simulink model "Example_Faulty_DataGen"  (R2022b)
settings: Solver=ode45  StartTime=0.0  StopTime=m_steps  FixedStep=ts  MaxStep=0.1  RelTol=1e-3  EnableMultiTasking=on
values from neighbouring files (symbols this model uses):
  A = 154    [init_model.m]
  a01 = 0.05    [init_model.m]
  a02 = 0.05    [init_model.m]
  attack_time = 70000    [fault_scenario.m]
  az1 = 0.46    [init_model.m]
  az2 = 0.60    (= 0.6)    [init_model.m]
  az3 = 0.45    [init_model.m]
  F_leak1_gain = fault_gain    [fault_scenario.m]    (also in init_model.m = 0)
  F_leak1_time = fault_time    [fault_scenario.m]    (also in init_model.m = 0)
  F_leak2_gain = fault_gain    [fault_scenario.m]    (also in init_model.m = 0)
  F_leak2_time = fault_time    [fault_scenario.m]    (also in init_model.m = 0)
  F_leak3_gain = fault_gain    [fault_scenario.m]    (also in init_model.m = 0)
  F_leak3_time = fault_time    [fault_scenario.m]    (also in init_model.m = 0)
  F_plugg13_gain = fault_gain    [fault_scenario.m]    (also in init_model.m = 0)
  F_plugg13_time = fault_time    [fault_scenario.m]    (also in init_model.m = 0)
  F_plugg20_gain = fault_gain    [fault_scenario.m]    (also in init_model.m = 0)
  F_plugg20_time = fault_time    [fault_scenario.m]    (also in init_model.m = 0)
  F_plugg32_gain = fault_gain    [fault_scenario.m]    (also in init_model.m = 0)
  F_plugg32_time = fault_time    [fault_scenario.m]    (also in init_model.m = 0)
  F_pump1_gain = fault_gain    [fault_scenario.m]    (also in init_model.m = 100)
  F_pump1_time = fault_time    [fault_scenario.m]    (also in init_model.m = 0)
  F_pump2_gain = fault_gain    [fault_scenario.m]    (also in init_model.m = 100)
  F_pump2_time = fault_time    [fault_scenario.m]    (also in init_model.m = 0)
  F_sensor1_offset = fault_gain    [fault_scenario.m]    (also in init_model.m = 0)
  F_sensor1_time = fault_time    [fault_scenario.m]    (also in init_model.m = 0)
  F_sensor2_offset = fault_gain    [fault_scenario.m]    (also in init_model.m = 0)
  F_sensor2_time = fault_time    [fault_scenario.m]    (also in init_model.m = 0)
  F_sensor3_offset = fault_gain    [fault_scenario.m]    (also in init_model.m = 0)
  F_sensor3_time = fault_time    [fault_scenario.m]    (also in init_model.m = 0)
  g = 981    [init_model.m]
  Hmax = 62    [init_model.m]
  l1 = a01    (= 0.05)    [init_model.m]
  l2 = a02    (= 0.05)    [init_model.m]
  m_ramp1 = 3e-4    (= 0.0003)    [fault_scenario.m]
  m_ramp2 = 0    [fault_scenario.m]
  m_satu = 1    [fault_scenario.m]
  m_satu1 = 460    [fault_scenario.m]
  m_satu2 = 160    [fault_scenario.m]
  m_satu3 = 320    [fault_scenario.m]
  m_ts = 2    [init_model.m]
  m_var1 = 0.2027    [init_model.m]
  m_var2 = 0.4394    [init_model.m]
  m_var3 = 0.0051    [init_model.m]
  p = s    [Att.m]    (also in init_model.m = 0)
  Q1max = 100    [init_model.m]
  Q2max = 100    [init_model.m]
  Sl = 0.5    [init_model.m]
  Sn = 0.5    [init_model.m]
  T_attack = 1000/(2*pi)    (= 159.154943092)    [fault_scenario.m]
  v = k    (= 0.0125)    [init_model.m]
libraries: simulink x5
settings Model: Creator=luo  LastModifiedBy=DaiQi Yang
settings SolverCC: AlgebraicLoopSolver=TrustRegion
settings DataIOCC: LimitDataPoints=on  SaveFormat=Array  SignalLoggingSaveFormat=ModelDataLogs  ReturnWorkspaceOutputs=off
settings OptimizationCC: ReuseModelBlockBuffer=on  ExpressionDepthLimit=2147483647  LifeSpan=inf
settings DebuggingCC: UnderspecifiedInitializationDetection=Classic  MergeDetectMultiDrivingBlocksExec=none  SolverPrmCheckMsg=warning  FcnCallInpInsideContextMsg=warning  UnconnectedInputMsg=warning  UnconnectedOutputMsg=warning  UnconnectedLineMsg=warning  StateNameClashWarn=warning  SFUnexpectedBacktrackingDiag=warning  SFNoUnconditionalDefaultTransitionDiag=warning  SFExecutionAtInitializationDiag=none  ArithmeticOperatorsInVariantConditions=warning
settings HardwareCC: ProdBitPerPointer=32  ProdBitPerSizeT=32  ProdBitPerPtrDiffT=32  ProdLargestAtomicFloat=None  ProdIntDivRoundTo=Undefined  ProdEndianess=Unspecified  ProdWordSize=32  ProdHWDeviceType=32-bit Generic
settings ModelReferenceCC: EnableRefExpFcnMdlSchedulingChecks=on  PropagateSignalLabelsOutOfModel=off
settings SFSimCC: SimUseLocalCustomCode=off  CustomCodeUndefinedFunction=UseInterfaceOnly
settings RTWCC: RTWUseLocalCustomCode=off
settings CodeAppCC: StateflowObjectComments=on
settings GRTTargetCC: TargetLangStandard=C89/C90 (ANSI)  CombineOutputUpdateFcns=off  GRTInterface=on
settings ConfigComp: CovMetricSettings=dw  CovSaveCumulativeToWorkspaceVar=on  CovSaveSingleToWorkspaceVar=on  CovExternalEMLEnable=off

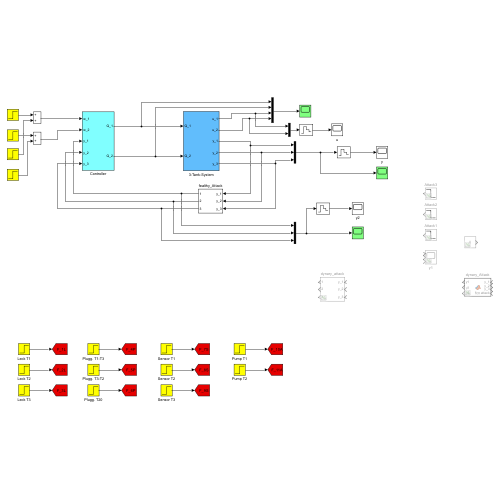
[thumbnail: Simulink's stored preview of the top-level diagram]
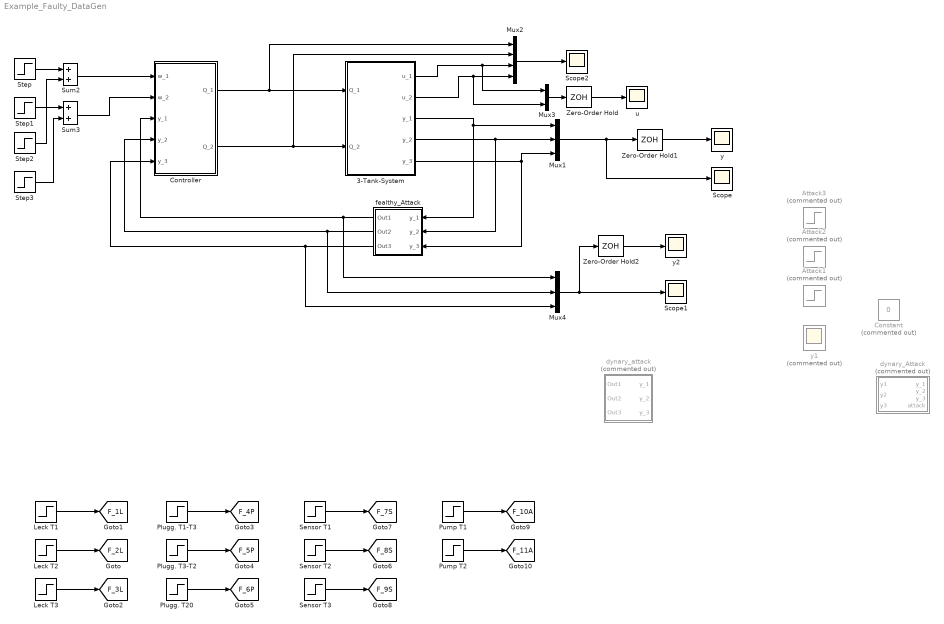
== system Example_Faulty_DataGen ==
  3-Tank-System : Subsystem
  Attack1 : Step  Commented=on  Time=attack_time  After=-0.352325574028282  SampleTime=0
  Attack2 : Step  Commented=on  Time=attack_time  After=-0.352325574028282  SampleTime=0
  Attack3 : Step  Commented=on  Time=attack_time  After=-0.352325574028282  SampleTime=0
  Constant : Constant  Commented=on  Value=0
  Controller : Subsystem
  Leck T1 : Step  Time=F_leak1_time  After=F_leak1_gain  SampleTime=0
  Leck T2 : Step  Time=F_leak2_time  After=F_leak2_gain  SampleTime=0
  Leck T3 : Step  Time=F_leak3_time  After=F_leak3_gain  SampleTime=0
  Mux1 : Mux  Inputs=3
  Mux2 : Mux
  Mux3 : Mux  Inputs=2
  Mux4 : Mux  Inputs=3
  Plugg. T1-T3 : Step  Time=F_plugg13_time  After=F_plugg13_gain  SampleTime=0
  Plugg. T20 : Step  Time=F_plugg20_time  After=F_plugg20_gain  SampleTime=0
  Plugg. T3-T2 : Step  Time=F_plugg32_time  After=F_plugg32_gain  SampleTime=0
  Pump T1 : Step  Time=F_pump1_time  Before=100  After=F_pump1_gain  SampleTime=0
  Pump T2 : Step  Time=F_pump2_time  Before=100  After=F_pump2_gain  SampleTime=0
  Scope : Scope
  Scope1 : Scope
  Scope2 : Scope
  Sensor T1 : Step  Time=500  Before=100  After=100  SampleTime=0
  Sensor T2 : Step  Time=500  Before=100  After=100  SampleTime=0
  Sensor T3 : Step  Time=500  Before=100  After=100  SampleTime=0
  Step : Step  Time=0  After=45  SampleTime=0
  Step1 : Step  Time=0  After=15  SampleTime=0
  Step2 : Step  Time=500  After=0  SampleTime=0
  Step3 : Step  Time=800  After=0  SampleTime=0
  Sum2 : Sum  SaturateOnIntegerOverflow=on
  Sum3 : Sum  SaturateOnIntegerOverflow=on
  Zero-Order Hold : ZeroOrderHold  SampleTime=m_ts
  Zero-Order Hold1 : ZeroOrderHold  SampleTime=m_ts
  Zero-Order Hold2 : ZeroOrderHold  SampleTime=m_ts
  dynary_Attack : MATLAB Function  Commented=on  TreatAsAtomicUnit=on
  dynary_attack : Subsystem  Commented=on
  fealthy_Attack : Subsystem
  u : Scope
  y : Scope
  y1 : Scope  Commented=on  NumInputPorts=3
  y2 : Scope
  tag scope: F_10A=global, F_11A=global, F_1L=global, F_2L=global, F_3L=global, F_4P=global, F_5P=global, F_6P=global, F_7S=global, F_8S=global, F_9S=global
  wires:
  Step/1 -> Sum2/1
  Step1/1 -> Sum3/1
  Step2/1 -> Sum2/2
  Step3/1 -> Sum3/2
  Mux1/1 -> Scope/1, Zero-Order Hold1/1
  Leck T2/1 -> [F_2L]
  Sum2/1 -> Controller/1(w_1)
  Leck T1/1 -> [F_1L]
  Leck T3/1 -> [F_3L]
  Plugg. T1-T3/1 -> [F_4P]
  Plugg. T3-T2/1 -> [F_5P]
  Plugg. T20/1 -> [F_6P]
  Sensor T2/1 -> [F_8S]
  Sensor T1/1 -> [F_7S]
  Sensor T3/1 -> [F_9S]
  Pump T1/1 -> [F_10A]
  Pump T2/1 -> [F_11A]
  Mux2/1 -> Scope2/1
  3-Tank-System/1(u_1) -> Mux3/1, Mux2/3
  3-Tank-System/2(u_2) -> Mux3/2, Mux2/4
  Controller/1(Q_1) -> 3-Tank-System/1(Q_1), Mux2/1
  Controller/2(Q_2) -> 3-Tank-System/2(Q_2), Mux2/2
  Sum3/1 -> Controller/2(w_2)
  Zero-Order Hold/1 -> u/1
  Zero-Order Hold1/1 -> y/1
  Mux3/1 -> Zero-Order Hold/1
  3-Tank-System/3(y_1) -> fealthy_Attack/1(y_1), Mux1/1
  3-Tank-System/4(y_2) -> fealthy_Attack/2(y_2), Mux1/2
  3-Tank-System/5(y_3) -> fealthy_Attack/3(y_3), Mux1/3
  fealthy_Attack/1(Out1) -> Mux4/1, Controller/3(y_1)
  fealthy_Attack/2(Out2) -> Mux4/2, Controller/4(y_2)
  fealthy_Attack/3(Out3) -> Mux4/3, Controller/5(y_3)
  Mux4/1 -> Scope1/1, Zero-Order Hold2/1
  Zero-Order Hold2/1 -> y2/1

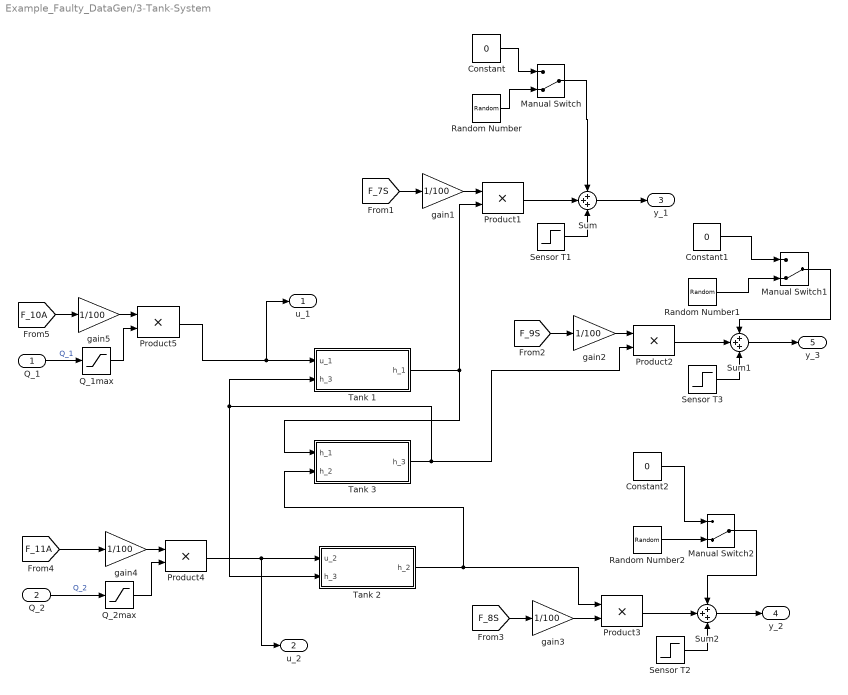
== system Example_Faulty_DataGen/3-Tank-System ==
  Q_1 : Inport
  Q_2 : Inport  Port=2
  Constant : Constant  Value=0
  Constant1 : Constant  Value=0
  Constant2 : Constant  Value=0
  Manual Switch : ManualSwitch  CurrentSetting=0
  Manual Switch1 : ManualSwitch  CurrentSetting=0
  Manual Switch2 : ManualSwitch  CurrentSetting=0
  Product{1..5} (5 alike) : Product  SaturateOnIntegerOverflow=on  OutDataTypeStr=Inherit: Same as first input
  Q_1max : Saturate  UpperLimit=Q1max  LowerLimit=0
  Q_2max : Saturate  UpperLimit=Q2max  LowerLimit=0
  Random Number : RandomNumber  Variance=m_var1  Seed=floor(1000*rand(1))  SampleTime=0
  Random Number1 : RandomNumber  Variance=m_var3  Seed=floor(1000*rand(1))  SampleTime=0
  Random Number2 : RandomNumber  Variance=m_var2  Seed=floor(1000*rand(1))  SampleTime=0
  Sensor T1 : Step  Time=F_sensor1_time  After=F_sensor1_offset  SampleTime=0
  Sensor T2 : Step  Time=F_sensor2_time  After=F_sensor2_offset  SampleTime=0
  Sensor T3 : Step  Time=F_sensor3_time  After=F_sensor3_offset  SampleTime=0
  Sum : Sum  Inputs=+++
  Sum1 : Sum  Inputs=+++
  Sum2 : Sum  Inputs=+++
  Tank 1 : Subsystem
  Tank 2 : Subsystem
  Tank 3 : Subsystem
  gain{1..5} (5 alike) : Gain  Gain=1/100  SaturateOnIntegerOverflow=on  OutDataTypeStr=Inherit: Same as input  ParamDataTypeStr=Inherit: Same as input
  u_1 : Outport  VectorParamsAs1DForOutWhenUnconnected=off
  u_2 : Outport  Port=2  VectorParamsAs1DForOutWhenUnconnected=off
  y_1 : Outport  Port=3  VectorParamsAs1DForOutWhenUnconnected=off
  y_2 : Outport  Port=4  VectorParamsAs1DForOutWhenUnconnected=off
  y_3 : Outport  Port=5  VectorParamsAs1DForOutWhenUnconnected=off
  wires:
  Tank 1/1(h_1) -> Tank 3/1(h_1), Product1/2
  Tank 3/1(h_3) -> Tank 1/2(h_3), Tank 2/2(h_3), Product2/2
  Tank 2/1(h_2) -> Tank 3/2(h_2), Product3/1
  [F_8S] -> gain3/1
  gain3/1 -> Product3/2
  gain1/1 -> Product1/1
  [F_7S] -> gain1/1
  gain2/1 -> Product2/1
  [F_9S] -> gain2/1
  gain4/1 -> Product4/1
  [F_11A] -> gain4/1
  Q_2/1 -> Q_2max/1  "Q_2"
  Product4/1 -> Tank 2/1(u_2), u_2/1
  gain5/1 -> Product5/1
  [F_10A] -> gain5/1
  Q_1/1 -> Q_1max/1  "Q_1"
  Product5/1 -> Tank 1/1(u_1), u_1/1
  Q_1max/1 -> Product5/2
  Q_2max/1 -> Product4/2
  Product1/1 -> Sum/2
  Sum/1 -> y_1/1
  Product2/1 -> Sum1/2
  Sum1/1 -> y_3/1
  Product3/1 -> Sum2/2
  Sum2/1 -> y_2/1
  Sensor T1/1 -> Sum/3
  Sensor T2/1 -> Sum2/3
  Sensor T3/1 -> Sum1/3
  Constant/1 -> Manual Switch/1
  Random Number/1 -> Manual Switch/2
  Manual Switch/1 -> Sum/1
  Random Number2/1 -> Manual Switch2/2
  Manual Switch2/1 -> Sum2/1
  Random Number1/1 -> Manual Switch1/2
  Manual Switch1/1 -> Sum1/1
  Constant1/1 -> Manual Switch1/1
  Constant2/1 -> Manual Switch2/1

== system Example_Faulty_DataGen/Controller ==
  w_1 : Inport
  w_2 : Inport  Port=2
  y_1 : Inport  Port=3
  y_2 : Inport  Port=4
  y_3 : Inport  Port=5
  Matrix F : Subsystem
  Matrix G : Subsystem
  PI controller 1 : Subsystem
  PI controller 2 : Subsystem
  Sum : Sum  Inputs=|+-
  Sum1 : Sum  Inputs=|+-
  Sum4 : Sum  SaturateOnIntegerOverflow=on
  Sum5 : Sum  SaturateOnIntegerOverflow=on
  Q_1 : Outport  VectorParamsAs1DForOutWhenUnconnected=off
  Q_2 : Outport  Port=2  VectorParamsAs1DForOutWhenUnconnected=off
  wires:
  Sum/1 -> PI controller 1/1(In1)
  Sum1/1 -> PI controller 2/1(In1)
  Matrix F/1(F_2) -> Sum4/2
  Matrix F/2(F_1) -> Sum5/2
  Matrix G/1(G_1) -> Sum5/1
  Matrix G/2(G_2) -> Sum4/1
  PI controller 1/1(Out1) -> Matrix G/1(w_1)
  PI controller 2/1(Out1) -> Matrix G/2(w_2)
  y_3/1 -> Matrix F/3(y_3)
  w_1/1 -> Sum/1
  Sum5/1 -> Q_1/1
  w_2/1 -> Sum1/1
  Sum4/1 -> Q_2/1
  y_2/1 -> Sum1/2, Matrix F/2(y_2)
  y_1/1 -> Matrix F/1(y_1), Sum/2

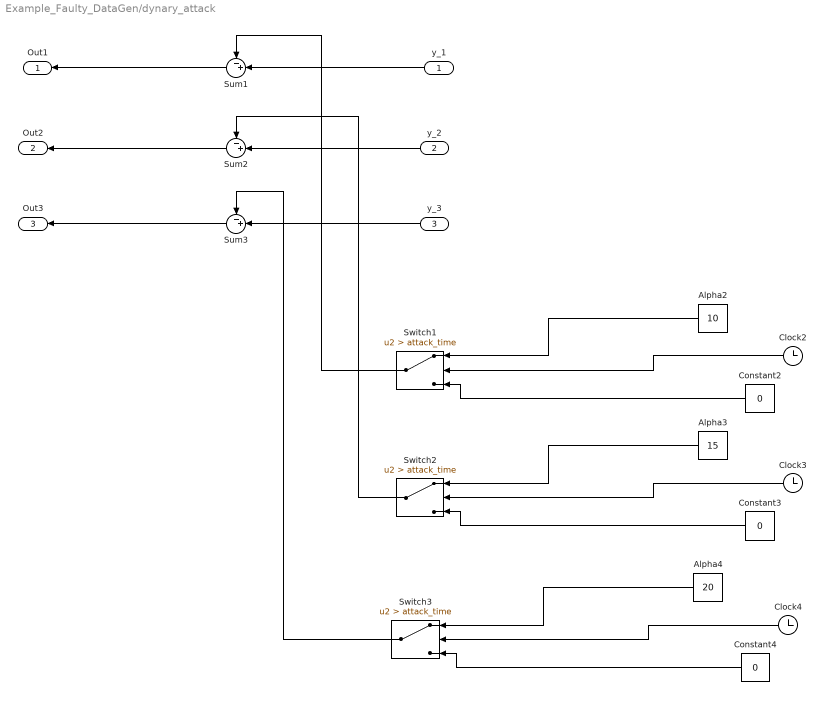
== system Example_Faulty_DataGen/dynary_attack ==
  y_1 : Inport
  y_2 : Inport  Port=2
  y_3 : Inport  Port=3
  Alpha2 : Constant  Value=10
  Alpha3 : Constant  Value=15
  Alpha4 : Constant  Value=20
  Clock2 : Clock
  Clock3 : Clock
  Clock4 : Clock
  Constant2 : Constant  Value=0
  Constant3 : Constant  Value=0
  Constant4 : Constant  Value=0
  Sum1 : Sum  Inputs=-+|
  Sum2 : Sum  Inputs=-+|
  Sum3 : Sum  Inputs=-+|
  Switch1 : Switch  Criteria=u2 > Threshold  Threshold=attack_time  SaturateOnIntegerOverflow=off  InputSameDT=off
  Switch2 : Switch  Criteria=u2 > Threshold  Threshold=attack_time  SaturateOnIntegerOverflow=off  InputSameDT=off
  Switch3 : Switch  Criteria=u2 > Threshold  Threshold=attack_time  SaturateOnIntegerOverflow=off  InputSameDT=off
  Out1 : Outport
  Out2 : Outport  Port=2
  Out3 : Outport  Port=3
  wires:
  Sum1/1 -> Out1/1
  y_1/1 -> Sum1/2
  Clock2/1 -> Switch1/2
  Constant2/1 -> Switch1/3
  Alpha2/1 -> Switch1/1
  Alpha3/1 -> Switch2/1
  Clock3/1 -> Switch2/2
  Constant3/1 -> Switch2/3
  Alpha4/1 -> Switch3/1
  Switch3/1 -> Sum3/1
  Clock4/1 -> Switch3/2
  Constant4/1 -> Switch3/3
  Sum2/1 -> Out2/1
  y_2/1 -> Sum2/2
  Sum3/1 -> Out3/1
  y_3/1 -> Sum3/2
  Switch1/1 -> Sum1/1
  Switch2/1 -> Sum2/1

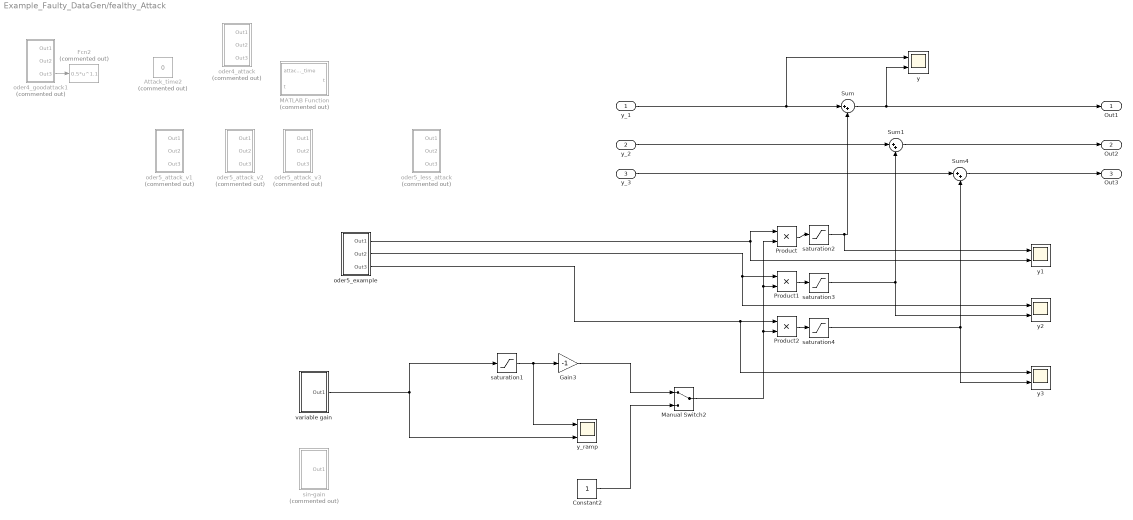
== system Example_Faulty_DataGen/fealthy_Attack ==
  y_1 : Inport
  y_2 : Inport  Port=2
  y_3 : Inport  Port=3
  Attack_time2 : Constant  Commented=on  Value=0
  Constant2 : Constant
  Fcn2 : Fcn  Commented=on  Expr=0.5*u^1.1
  Gain3 : Gain  Gain=-1
  MATLAB Function : MATLAB Function  Commented=on  TreatAsAtomicUnit=on
  Manual Switch2 : ManualSwitch
  Product : Product
  Product1 : Product
  Product2 : Product
  Sum : Sum  Inputs=|++
  Sum1 : Sum  Inputs=|++
  Sum4 : Sum  Inputs=|++
  oder4_attack : Subsystem  Commented=on
  oder4_goodattack1 : Subsystem  Commented=on
  oder5_attack_v1 : Subsystem  Commented=on
  oder5_attack_v2 : Subsystem  Commented=on
  oder5_attack_v3 : Subsystem  Commented=on
  oder5_example : Subsystem
  oder5_less_attack : Subsystem  Commented=on
  saturation1 : Saturate  UpperLimit=m_satu  LowerLimit=-m_satu
  saturation2 : Saturate  UpperLimit=m_satu1  LowerLimit=-m_satu1
  saturation3 : Saturate  UpperLimit=m_satu2  LowerLimit=-m_satu2
  saturation4 : Saturate  UpperLimit=m_satu3  LowerLimit=-m_satu3
  sin-gain : Subsystem  Commented=on
  variable gain : Subsystem
  y{,1..3} (4 alike) : Scope  NumInputPorts=2
  y_ramp : Scope  NumInputPorts=2
  Out1 : Outport
  Out2 : Outport  Port=2
  Out3 : Outport  Port=3
  wires:
  Sum/1 -> y/2, Out1/1
  y_1/1 -> y/1, Sum/1
  Sum4/1 -> Out3/1
  Sum1/1 -> Out2/1
  y_3/1 -> Sum4/1
  y_2/1 -> Sum1/1
  Product/1 -> saturation2/1
  saturation1/1 -> y_ramp/1, Gain3/1
  Constant2/1 -> Manual Switch2/2
  Manual Switch2/1 -> Product2/2, Product1/2, Product/2
  Gain3/1 -> Manual Switch2/1
  saturation2/1 -> y1/1, Sum/2
  Product1/1 -> saturation3/1
  saturation3/1 -> y2/2, Sum1/2
  Product2/1 -> saturation4/1
  saturation4/1 -> Sum4/2, y3/2
  oder5_example/1(Out1) -> y1/2, Product/1
  oder5_example/2(Out2) -> y2/1, Product1/1
  oder5_example/3(Out3) -> y3/1, Product2/1
  variable gain/1(Out1) -> saturation1/1, y_ramp/2
  oder4_goodattack1/3(Out3) -> Fcn2/1

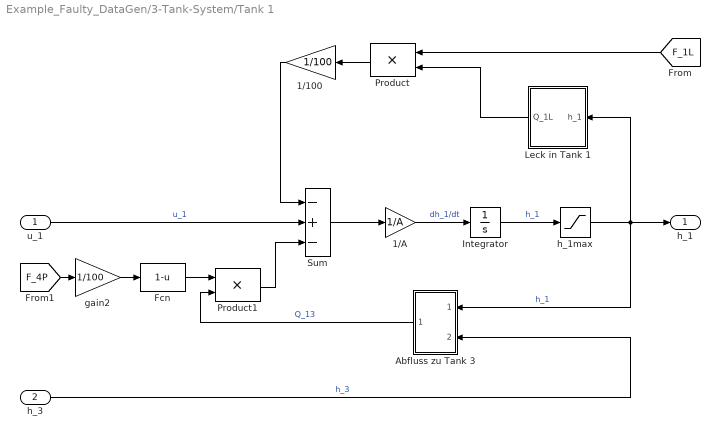
== system Example_Faulty_DataGen/3-Tank-System/Tank 1 ==
  u_1 : Inport
  h_3 : Inport  Port=2
  1/100 : Gain  Gain=1/100  SaturateOnIntegerOverflow=on  OutDataTypeStr=Inherit: Same as input  ParamDataTypeStr=Inherit: Same as input
  1/A : Gain  Gain=1/A  SaturateOnIntegerOverflow=on  OutDataTypeStr=Inherit: Same as input  ParamDataTypeStr=Inherit: Same as input
  Abfluss zu Tank 3 : Subsystem
  Fcn : Fcn  Expr=1-u
  Integrator : Integrator  InitialCondition=0.3
  Leck in Tank 1 : Subsystem
  Product : Product  SaturateOnIntegerOverflow=on  OutDataTypeStr=Inherit: Same as first input
  Product1 : Product  SaturateOnIntegerOverflow=on  OutDataTypeStr=Inherit: Same as first input
  Sum : Sum  Inputs=-+-  SaturateOnIntegerOverflow=on
  gain2 : Gain  Gain=1/100  SaturateOnIntegerOverflow=on  OutDataTypeStr=Inherit: Same as input  ParamDataTypeStr=Inherit: Same as input
  h_1max : Saturate  UpperLimit=Hmax  LowerLimit=0
  h_1 : Outport  VectorParamsAs1DForOutWhenUnconnected=off
  wires:
  1/A/1 -> Integrator/1  "dh_1/dt"
  h_1max/1 -> Abfluss zu Tank 3/1(h_1), Leck in Tank 1/1(h_1), h_1/1  "h_1"
  Integrator/1 -> h_1max/1  "h_1"
  Sum/1 -> 1/A/1
  h_3/1 -> Abfluss zu Tank 3/2(h_3)  "h_3"
  Product/1 -> 1/100/1
  [F_1L] -> Product/1
  Product1/1 -> Sum/3
  Abfluss zu Tank 3/1(Q_13) -> Product1/2  "Q_13"
  1/100/1 -> Sum/1
  Leck in Tank 1/1(Q_1L) -> Product/2
  gain2/1 -> Fcn/1
  [F_4P] -> gain2/1
  Fcn/1 -> Product1/1
  u_1/1 -> Sum/2  "u_1"

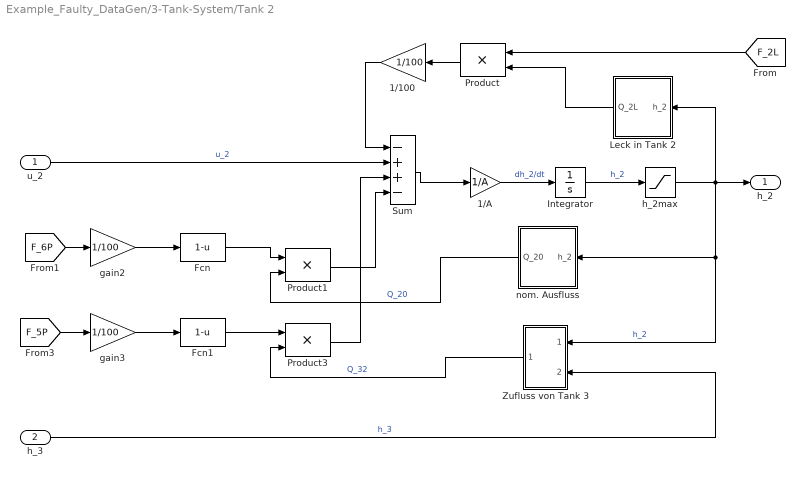
== system Example_Faulty_DataGen/3-Tank-System/Tank 2 ==
  u_2 : Inport
  h_3 : Inport  Port=2
  1/100 : Gain  Gain=1/100  SaturateOnIntegerOverflow=on  OutDataTypeStr=Inherit: Same as input  ParamDataTypeStr=Inherit: Same as input
  1/A : Gain  Gain=1/A  SaturateOnIntegerOverflow=on  OutDataTypeStr=Inherit: Same as input  ParamDataTypeStr=Inherit: Same as input
  Fcn : Fcn  Expr=1-u
  Fcn1 : Fcn  Expr=1-u
  Integrator : Integrator  InitialCondition=0.2
  Leck in Tank 2 : Subsystem
  Product : Product  SaturateOnIntegerOverflow=on  OutDataTypeStr=Inherit: Same as first input
  Product1 : Product  SaturateOnIntegerOverflow=on  OutDataTypeStr=Inherit: Same as first input
  Product3 : Product  SaturateOnIntegerOverflow=on  OutDataTypeStr=Inherit: Same as first input
  Sum : Sum  Inputs=-++-  SaturateOnIntegerOverflow=on
  Zufluss von Tank 3 : Subsystem
  gain2 : Gain  Gain=1/100  SaturateOnIntegerOverflow=on  OutDataTypeStr=Inherit: Same as input  ParamDataTypeStr=Inherit: Same as input
  gain3 : Gain  Gain=1/100  SaturateOnIntegerOverflow=on  OutDataTypeStr=Inherit: Same as input  ParamDataTypeStr=Inherit: Same as input
  h_2max : Saturate  UpperLimit=Hmax  LowerLimit=0
  nom. Ausfluss : Subsystem
  h_2 : Outport  VectorParamsAs1DForOutWhenUnconnected=off
  wires:
  1/A/1 -> Integrator/1  "dh_2/dt"
  h_2max/1 -> nom. Ausfluss/1(h_2), Zufluss von Tank 3/1(h_1), Leck in Tank 2/1(h_2), h_2/1  "h_2"
  Integrator/1 -> h_2max/1  "h_2"
  Sum/1 -> 1/A/1
  h_3/1 -> Zufluss von Tank 3/2(h_3)  "h_3"
  Product/1 -> 1/100/1
  [F_2L] -> Product/1
  1/100/1 -> Sum/1
  Leck in Tank 2/1(Q_2L) -> Product/2
  gain2/1 -> Fcn/1
  [F_6P] -> gain2/1
  gain3/1 -> Fcn1/1
  [F_5P] -> gain3/1
  nom. Ausfluss/1(Q_20) -> Product1/2  "Q_20"
  Product1/1 -> Sum/4
  Zufluss von Tank 3/1(Q_32) -> Product3/2  "Q_32"
  Product3/1 -> Sum/3
  Fcn/1 -> Product1/1
  Fcn1/1 -> Product3/1
  u_2/1 -> Sum/2  "u_2"

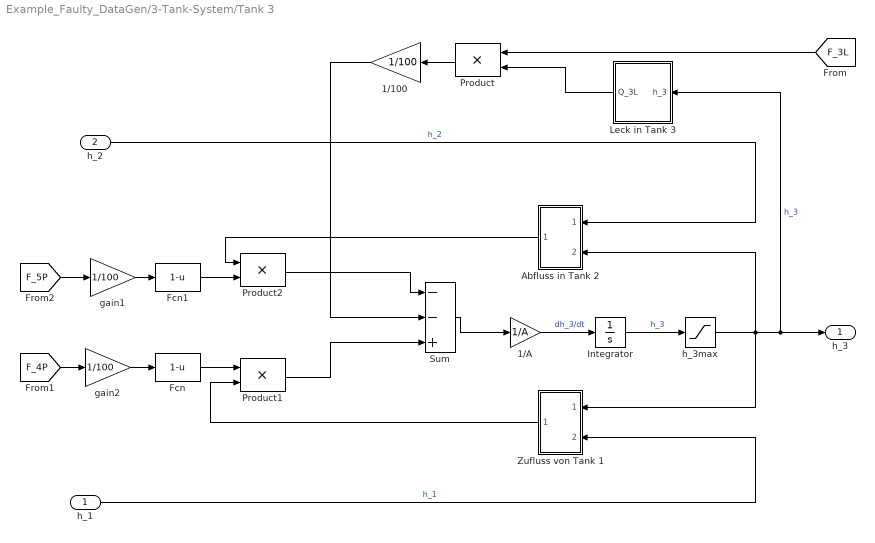
== system Example_Faulty_DataGen/3-Tank-System/Tank 3 ==
  h_1 : Inport
  h_2 : Inport  Port=2
  1/100 : Gain  Gain=1/100  SaturateOnIntegerOverflow=on  OutDataTypeStr=Inherit: Same as input  ParamDataTypeStr=Inherit: Same as input
  1/A : Gain  Gain=1/A  SaturateOnIntegerOverflow=on  OutDataTypeStr=Inherit: Same as input  ParamDataTypeStr=Inherit: Same as input
  Abfluss in Tank 2 : Subsystem
  Fcn : Fcn  Expr=1-u
  Fcn1 : Fcn  Expr=1-u
  Integrator : Integrator  InitialCondition=0.25
  Leck in Tank 3 : Subsystem
  Product : Product  SaturateOnIntegerOverflow=on  OutDataTypeStr=Inherit: Same as first input
  Product1 : Product  SaturateOnIntegerOverflow=on  OutDataTypeStr=Inherit: Same as first input
  Product2 : Product  SaturateOnIntegerOverflow=on  OutDataTypeStr=Inherit: Same as first input
  Sum : Sum  Inputs=--+  SaturateOnIntegerOverflow=on
  Zufluss von Tank 1 : Subsystem
  gain1 : Gain  Gain=1/100  SaturateOnIntegerOverflow=on  OutDataTypeStr=Inherit: Same as input  ParamDataTypeStr=Inherit: Same as input
  gain2 : Gain  Gain=1/100  SaturateOnIntegerOverflow=on  OutDataTypeStr=Inherit: Same as input  ParamDataTypeStr=Inherit: Same as input
  h_3max : Saturate  UpperLimit=Hmax  LowerLimit=0
  h_3 : Outport  VectorParamsAs1DForOutWhenUnconnected=off
  wires:
  1/A/1 -> Integrator/1  "dh_3/dt"
  h_3max/1 -> Abfluss in Tank 2/2(h_3), Zufluss von Tank 1/1(h_3), h_3/1, Leck in Tank 3/1(h_3)  "h_3"
  Integrator/1 -> h_3max/1  "h_3"
  Sum/1 -> 1/A/1
  h_1/1 -> Zufluss von Tank 1/2(h_1)  "h_1"
  h_2/1 -> Abfluss in Tank 2/1(h_2)  "h_2"
  Product/1 -> 1/100/1
  [F_3L] -> Product/1
  gain2/1 -> Fcn/1
  [F_4P] -> gain2/1
  [F_5P] -> gain1/1
  1/100/1 -> Sum/2
  Leck in Tank 3/1(Q_3L) -> Product/2
  Abfluss in Tank 2/1(Q_32) -> Product2/1
  gain1/1 -> Fcn1/1
  Product2/1 -> Sum/1
  Zufluss von Tank 1/1(Q_13) -> Product1/2
  Product1/1 -> Sum/3
  Fcn/1 -> Product1/1
  Fcn1/1 -> Product2/2

== system Example_Faulty_DataGen/Controller/Matrix F ==
  y_1 : Inport
  y_2 : Inport  Port=2
  y_3 : Inport  Port=3
  Abfluss in Tank 2 : Subsystem
  Abfluss zu Tank 3 : Subsystem
  Gain : Gain  Gain=A*a01  SaturateOnIntegerOverflow=on  OutDataTypeStr=Inherit: Same as input  ParamDataTypeStr=Inherit: Same as input
  Gain2 : Gain  Gain=A*a02  SaturateOnIntegerOverflow=on  OutDataTypeStr=Inherit: Same as input  ParamDataTypeStr=Inherit: Same as input
  Sum : Sum  Inputs=-+-  SaturateOnIntegerOverflow=on
  Sum1 : Sum  Inputs=-+  SaturateOnIntegerOverflow=on
  nom. Ausfluss : Subsystem
  F_2 : Outport  VectorParamsAs1DForOutWhenUnconnected=off
  F_1 : Outport  Port=2  VectorParamsAs1DForOutWhenUnconnected=off
  wires:
  y_1/1 -> Abfluss zu Tank 3/1(h_1), Gain/1
  y_3/1 -> Abfluss in Tank 2/1(h_3), Abfluss zu Tank 3/2(h_3)
  y_2/1 -> nom. Ausfluss/1(h_2), Abfluss in Tank 2/2(h_2), Gain2/1
  Sum1/1 -> F_1/1
  Gain/1 -> Sum1/1
  Abfluss zu Tank 3/1(Q_13) -> Sum1/2
  Abfluss in Tank 2/1(Q_32) -> Sum/1
  nom. Ausfluss/1(Q_20) -> Sum/2
  Gain2/1 -> Sum/3
  Sum/1 -> F_2/1

== system Example_Faulty_DataGen/Controller/Matrix G ==
  w_1 : Inport
  w_2 : Inport  Port=2
  Gain 1 : Gain  Gain=A*l1
  Gain 2 : Gain  Gain=A*l2
  G_1 : Outport  VectorParamsAs1DForOutWhenUnconnected=off
  G_2 : Outport  Port=2  VectorParamsAs1DForOutWhenUnconnected=off
  wires:
  w_1/1 -> Gain 1/1
  Gain 1/1 -> G_1/1
  w_2/1 -> Gain 2/1
  Gain 2/1 -> G_2/1

== system Example_Faulty_DataGen/Controller/PI controller 1 ==
  In1 : Inport
  Int1 : Integrator  InitialCondition=0.4
  P1 : Gain  Gain=p
  Sum : Sum  Inputs=|++
  v=k : Gain  Gain=v
  Out1 : Outport  VectorParamsAs1DForOutWhenUnconnected=off
  wires:
  In1/1 -> v=k/1
  P1/1 -> Sum/2
  Int1/1 -> Sum/1
  Sum/1 -> Out1/1
  v=k/1 -> P1/1, Int1/1

== system Example_Faulty_DataGen/Controller/PI controller 2 ==
  In1 : Inport
  Int1 : Integrator  InitialCondition=0.2
  P1 : Gain  Gain=p
  Sum : Sum  Inputs=|++
  v=k : Gain  Gain=v
  Out1 : Outport  VectorParamsAs1DForOutWhenUnconnected=off
  wires:
  In1/1 -> v=k/1
  P1/1 -> Sum/2
  Int1/1 -> Sum/1
  Sum/1 -> Out1/1
  v=k/1 -> P1/1, Int1/1

== system Example_Faulty_DataGen/fealthy_Attack/oder4_attack ==
  Attack1 : Polyval  Coefs=|
      | [0.0147
      | -0.3439
      | 2.7873
      | -9.1137
      | 6.0715]
  Attack2 : Polyval  Coefs=|
      | [0.0187
      | -0.4361
      | 3.5079
      | -11.3885
      | 11.0519]
  Attack3 : Polyval  Coefs=|
      | [-0.0713
      | 1.6694
      | -13.5181
      | 44.1571
      | -50.2598]
  Attack_time : Constant  Value=attack_time
  Clock1 : Clock
  Clock2 : Clock
  Constant1 : Constant  Value=0
  Fcn3 : Fcn  Expr=rem(u,8)+2
  Sum2 : Sum  Inputs=-+|
  Switch : Switch  Criteria=u2 > Threshold  Threshold=attack_time  SaturateOnIntegerOverflow=off  InputSameDT=off
  Out1 : Outport
  Out2 : Outport  Port=2
  Out3 : Outport  Port=3
  wires:
  Fcn3/1 -> Attack3/1, Attack2/1, Attack1/1
  Constant1/1 -> Switch/3
  Clock1/1 -> Switch/2
  Clock2/1 -> Sum2/2
  Attack_time/1 -> Sum2/1
  Sum2/1 -> Switch/1
  Attack3/1 -> Out3/1
  Attack1/1 -> Out1/1
  Attack2/1 -> Out2/1
  Switch/1 -> Fcn3/1

== system Example_Faulty_DataGen/fealthy_Attack/oder4_goodattack1 ==
  Attack1 : Polyval  Coefs=|
      | [-0.0052
      | 0.1260
      | -1.1132
      | 4.2802
      | -6.0214]*10
  Attack2 : Polyval  Coefs=0
  Attack3 : Polyval  Coefs=|
      | [0.0001
      | -0.0022
      | 0.0203
      | -0.0733
      | 0.0820]*10
  Attack_time : Constant  Value=attack_time
  Clock1 : Clock
  Clock2 : Clock
  Constant1 : Constant  Value=0
  Fcn3 : Fcn  Expr=rem(u,8)+2
  Sum2 : Sum  Inputs=-+|
  Switch : Switch  Criteria=u2 > Threshold  Threshold=attack_time  SaturateOnIntegerOverflow=off  InputSameDT=off
  Out1 : Outport
  Out2 : Outport  Port=2
  Out3 : Outport  Port=3
  wires:
  Fcn3/1 -> Attack3/1, Attack2/1, Attack1/1
  Constant1/1 -> Switch/3
  Clock1/1 -> Switch/2
  Clock2/1 -> Sum2/2
  Attack_time/1 -> Sum2/1
  Sum2/1 -> Switch/1
  Attack3/1 -> Out3/1
  Attack1/1 -> Out1/1
  Attack2/1 -> Out2/1
  Switch/1 -> Fcn3/1

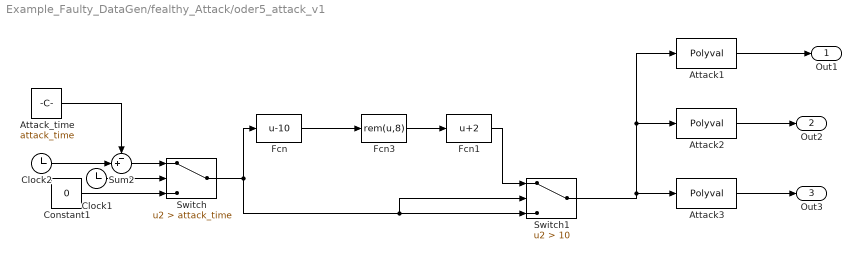
== system Example_Faulty_DataGen/fealthy_Attack/oder5_attack_v1 ==
  Attack1 : Polyval  Coefs=[0.0016,-0.0328,0.1937,-0.0587,-2.2821,0]
  Attack2 : Polyval  Coefs=|
      | [0.0029
      | -0.0676
      | 0.5425
      | -1.6727
      | 1.2291
      | 0.0000]
  Attack3 : Polyval  Coefs=|
      | [-0.0131
      | 0.3214
      | -2.7807
      | 10.0412
      | -13.2229
      | -0.0000]
  Attack_time : Constant  Value=attack_time
  Clock1 : Clock
  Clock2 : Clock
  Constant1 : Constant  Value=0
  Fcn : Fcn  Expr=u-10
  Fcn1 : Fcn  Expr=u+2
  Fcn3 : Fcn  Expr=rem(u,8)
  Sum2 : Sum  Inputs=-+|
  Switch : Switch  Criteria=u2 > Threshold  Threshold=attack_time  SaturateOnIntegerOverflow=off  InputSameDT=off
  Switch1 : Switch  Criteria=u2 > Threshold  Threshold=10  SaturateOnIntegerOverflow=off  InputSameDT=off
  Out1 : Outport
  Out2 : Outport  Port=2
  Out3 : Outport  Port=3
  wires:
  Switch1/1 -> Attack3/1, Attack2/1, Attack1/1
  Fcn1/1 -> Switch1/1
  Constant1/1 -> Switch/3
  Clock1/1 -> Switch/2
  Fcn/1 -> Fcn3/1
  Fcn3/1 -> Fcn1/1
  Clock2/1 -> Sum2/2
  Switch/1 -> Switch1/2, Switch1/3, Fcn/1
  Attack_time/1 -> Sum2/1
  Sum2/1 -> Switch/1
  Attack3/1 -> Out3/1
  Attack1/1 -> Out1/1
  Attack2/1 -> Out2/1

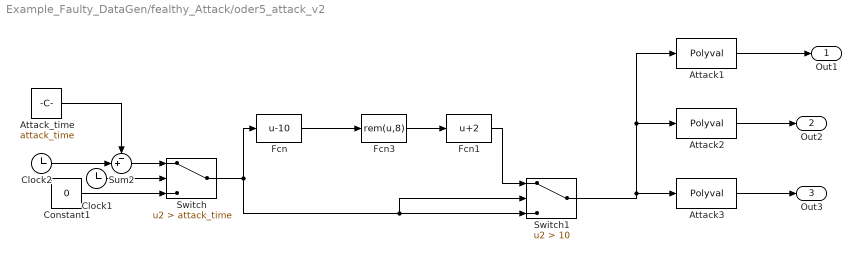
== system Example_Faulty_DataGen/fealthy_Attack/oder5_attack_v2 ==
  Attack1 : Polyval  Coefs=|
      | [-0.0055
      | 0.1400
      | -1.2612
      | 4.7911
      | -7.1804
      | -0.0000]
  Attack2 : Polyval  Coefs=|
      | [-0.0063
      | 0.1562
      | -1.3559
      | 4.7877
      | -6.0414
      | -0.0000]
  Attack3 : Polyval  Coefs=|
      | [0.0227
      | -0.5589
      | 4.7510
      | -15.9985
      | 17.2918
      | 0.0000]
  Attack_time : Constant  Value=attack_time
  Clock1 : Clock
  Clock2 : Clock
  Constant1 : Constant  Value=0
  Fcn : Fcn  Expr=u-10
  Fcn1 : Fcn  Expr=u+2
  Fcn3 : Fcn  Expr=rem(u,8)
  Sum2 : Sum  Inputs=-+|
  Switch : Switch  Criteria=u2 > Threshold  Threshold=attack_time  SaturateOnIntegerOverflow=off  InputSameDT=off
  Switch1 : Switch  Criteria=u2 > Threshold  Threshold=10  SaturateOnIntegerOverflow=off  InputSameDT=off
  Out1 : Outport
  Out2 : Outport  Port=2
  Out3 : Outport  Port=3
  wires:
  Switch1/1 -> Attack3/1, Attack2/1, Attack1/1
  Fcn1/1 -> Switch1/1
  Constant1/1 -> Switch/3
  Clock1/1 -> Switch/2
  Fcn/1 -> Fcn3/1
  Fcn3/1 -> Fcn1/1
  Clock2/1 -> Sum2/2
  Switch/1 -> Switch1/2, Switch1/3, Fcn/1
  Attack_time/1 -> Sum2/1
  Sum2/1 -> Switch/1
  Attack3/1 -> Out3/1
  Attack1/1 -> Out1/1
  Attack2/1 -> Out2/1

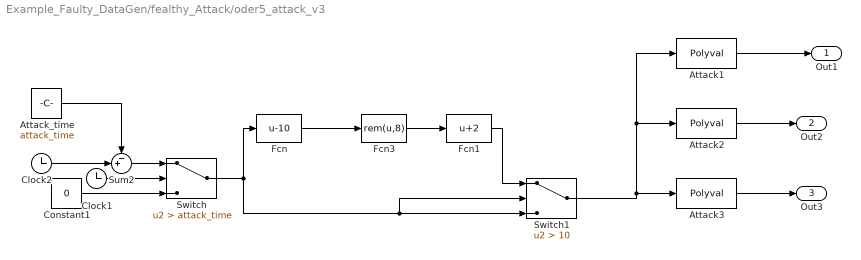
== system Example_Faulty_DataGen/fealthy_Attack/oder5_attack_v3 ==
  Attack1 : Polyval  Coefs=|
      | [0.0014
      | -0.0312
      | 0.2369
      | -0.7727
      | 0.9160
      | 0.0000]
  Attack2 : Polyval  Coefs=|
      | [0.0018
      | -0.0384
      | 0.2886
      | -0.9500
      | 1.1812
      | 0.0000]
  Attack3 : Polyval  Coefs=|
      | [-0.0068
      | 0.1461
      | -1.0905
      | 3.4223
      | -3.5299
      | -0.0000]
  Attack_time : Constant  Value=attack_time
  Clock1 : Clock
  Clock2 : Clock
  Constant1 : Constant  Value=0
  Fcn : Fcn  Expr=u-10
  Fcn1 : Fcn  Expr=u+2
  Fcn3 : Fcn  Expr=rem(u,8)
  Sum2 : Sum  Inputs=-+|
  Switch : Switch  Criteria=u2 > Threshold  Threshold=attack_time  SaturateOnIntegerOverflow=off  InputSameDT=off
  Switch1 : Switch  Criteria=u2 > Threshold  Threshold=10  SaturateOnIntegerOverflow=off  InputSameDT=off
  Out1 : Outport
  Out2 : Outport  Port=2
  Out3 : Outport  Port=3
  wires:
  Switch1/1 -> Attack3/1, Attack2/1, Attack1/1
  Fcn1/1 -> Switch1/1
  Constant1/1 -> Switch/3
  Clock1/1 -> Switch/2
  Fcn/1 -> Fcn3/1
  Fcn3/1 -> Fcn1/1
  Clock2/1 -> Sum2/2
  Switch/1 -> Switch1/2, Switch1/3, Fcn/1
  Attack_time/1 -> Sum2/1
  Sum2/1 -> Switch/1
  Attack3/1 -> Out3/1
  Attack1/1 -> Out1/1
  Attack2/1 -> Out2/1

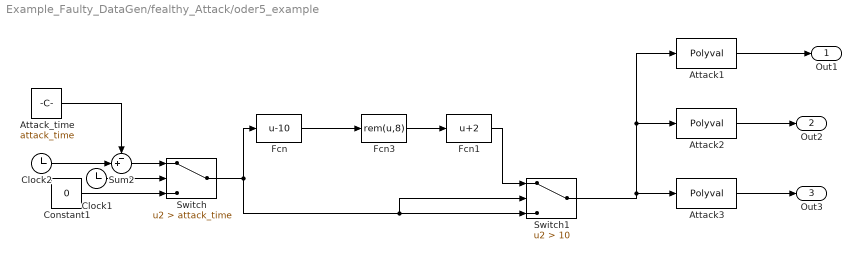
== system Example_Faulty_DataGen/fealthy_Attack/oder5_example ==
  Attack1 : Polyval  Coefs=|
      | [0.0051
      | -0.1298
      | 1.1774
      | -4.5904
      | 7.3440
      | 0.0000]
  Attack2 : Polyval  Coefs=|
      | [0.0056
      | -0.1386
      | 1.1968
      | -4.2593
      | 5.5835
      | 0.0000]
  Attack3 : Polyval  Coefs=|
      | [-0.0197
      | 0.4796
      | -4.0080
      | 13.2375
      | -13.6651
      | -0.0000]
  Attack_time : Constant  Value=attack_time
  Clock1 : Clock
  Clock2 : Clock
  Constant1 : Constant  Value=0
  Fcn : Fcn  Expr=u-10
  Fcn1 : Fcn  Expr=u+2
  Fcn3 : Fcn  Expr=rem(u,8)
  Sum2 : Sum  Inputs=-+|
  Switch : Switch  Criteria=u2 > Threshold  Threshold=attack_time  SaturateOnIntegerOverflow=off  InputSameDT=off
  Switch1 : Switch  Criteria=u2 > Threshold  Threshold=10  SaturateOnIntegerOverflow=off  InputSameDT=off
  Out1 : Outport
  Out2 : Outport  Port=2
  Out3 : Outport  Port=3
  wires:
  Switch1/1 -> Attack3/1, Attack2/1, Attack1/1
  Fcn1/1 -> Switch1/1
  Constant1/1 -> Switch/3
  Clock1/1 -> Switch/2
  Fcn/1 -> Fcn3/1
  Fcn3/1 -> Fcn1/1
  Clock2/1 -> Sum2/2
  Switch/1 -> Switch1/2, Switch1/3, Fcn/1
  Attack_time/1 -> Sum2/1
  Sum2/1 -> Switch/1
  Attack3/1 -> Out3/1
  Attack1/1 -> Out1/1
  Attack2/1 -> Out2/1

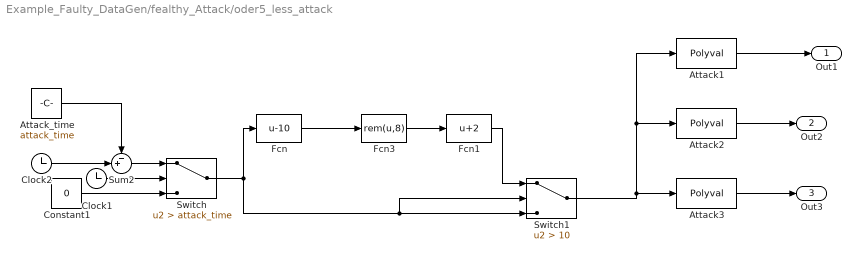
== system Example_Faulty_DataGen/fealthy_Attack/oder5_less_attack ==
  Attack1 : Polyval  Coefs=|
      | [-0.0013
      | 0.0385
      | -0.4128
      | 1.9220
      | -3.9722
      | -0.0000]
  Attack2 : Polyval  Coefs=|
      | [-0.0009
      | 0.0279
      | -0.2839
      | 1.1415
      | -1.8252
      | -0.0000]
  Attack3 : Polyval  Coefs=|
      | [0.0020
      | -0.0614
      | 0.5793
      | -1.7901
      | 1.0116
      | 0.0000]
  Attack_time : Constant  Value=attack_time
  Clock1 : Clock
  Clock2 : Clock
  Constant1 : Constant  Value=0
  Fcn : Fcn  Expr=u-10
  Fcn1 : Fcn  Expr=u+2
  Fcn3 : Fcn  Expr=rem(u,8)
  Sum2 : Sum  Inputs=-+|
  Switch : Switch  Criteria=u2 > Threshold  Threshold=attack_time  SaturateOnIntegerOverflow=off  InputSameDT=off
  Switch1 : Switch  Criteria=u2 > Threshold  Threshold=10  SaturateOnIntegerOverflow=off  InputSameDT=off
  Out1 : Outport
  Out2 : Outport  Port=2
  Out3 : Outport  Port=3
  wires:
  Switch1/1 -> Attack3/1, Attack2/1, Attack1/1
  Fcn1/1 -> Switch1/1
  Constant1/1 -> Switch/3
  Clock1/1 -> Switch/2
  Fcn/1 -> Fcn3/1
  Fcn3/1 -> Fcn1/1
  Clock2/1 -> Sum2/2
  Switch/1 -> Switch1/2, Switch1/3, Fcn/1
  Attack_time/1 -> Sum2/1
  Sum2/1 -> Switch/1
  Attack3/1 -> Out3/1
  Attack1/1 -> Out1/1
  Attack2/1 -> Out2/1

== system Example_Faulty_DataGen/fealthy_Attack/sin-gain ==
  Clock1 : Clock
  Sine Wave : Sin  Amplitude=0.1  Frequency=1/(2*T_attack)  SampleTime=0
  Sine Wave1 : Sin  Amplitude=0.01  Frequency=1/T_attack  SampleTime=0
  Sine Wave2 : Sin  Commented=on  Amplitude=0.2  Frequency=1/(3*T_attack)  SampleTime=0
  Sine Wave3 : Sin  Commented=on  Amplitude=0.1  Frequency=1/(2*T_attack)  SampleTime=0
  Sine Wave4 : Sin  Amplitude=0.1  Frequency=1/(2*T_attack)  SampleTime=0
  Switch : Switch  Criteria=u2 > Threshold  Threshold=attack_time+1000  SaturateOnIntegerOverflow=off  InputSameDT=off
  Switch1 : Switch  Criteria=u2 > Threshold  Threshold=attack_time+3000  SaturateOnIntegerOverflow=off  InputSameDT=off
  y_ramp1 : Scope  NumInputPorts=3
  y_ramp2 : Scope
  Out1 : Outport
  wires:
  Sine Wave4/1 -> y_ramp1/3, Switch/1
  Clock1/1 -> Switch1/2, Switch/2
  Sine Wave1/1 -> y_ramp1/1, Switch/3
  Sine Wave/1 -> y_ramp1/2, Switch1/1
  Switch/1 -> Switch1/3
  Switch1/1 -> y_ramp2/1, Out1/1

== system Example_Faulty_DataGen/fealthy_Attack/variable gain ==
  Ramp : simulink/Sources/Ramp  slope=m_ramp1  start=attack_time  InitialOutput=0
  Ramp1 : simulink/Sources/Ramp  slope=m_ramp2  start=attack_time+2000  InitialOutput=0
  Ramp2 : simulink/Sources/Ramp  slope=m_ramp2  start=attack_time+4000  InitialOutput=0
  Ramp3 : simulink/Sources/Ramp  slope=m_ramp2  start=attack_time+6000  InitialOutput=0
  Ramp4 : simulink/Sources/Ramp  slope=m_ramp2  start=attack_time+8000  InitialOutput=0
  Sum3 : Sum  Inputs=|+++++
  Out1 : Outport
  wires:
  Ramp1/1 -> Sum3/2
  Sum3/1 -> Out1/1
  Ramp3/1 -> Sum3/4
  Ramp/1 -> Sum3/1
  Ramp4/1 -> Sum3/5
  Ramp2/1 -> Sum3/3

== system Example_Faulty_DataGen/3-Tank-System/Tank 1/Abfluss zu Tank 3 ==
  h_1 : Inport
  h_3 : Inport  Port=2
  2*g : Gain  Gain=2*g  SaturateOnIntegerOverflow=on  OutDataTypeStr=Inherit: Same as input  ParamDataTypeStr=Inherit: Same as input
  Abs : Abs
  Math Function : Math  Operator=sqrt  SignedPower=on
  Product : Product  SaturateOnIntegerOverflow=on  OutDataTypeStr=Inherit: Same as first input
  Sign : Signum
  Sum1 : Sum  Inputs=+-  SaturateOnIntegerOverflow=on
  az_1*Sn : Gain  Gain=az1*Sn  SaturateOnIntegerOverflow=on  OutDataTypeStr=Inherit: Same as input  ParamDataTypeStr=Inherit: Same as input
  Q_13 : Outport  VectorParamsAs1DForOutWhenUnconnected=off
  wires:
  Sum1/1 -> Sign/1, Abs/1  "h_1-h_3"
  Sign/1 -> az_1*Sn/1
  Abs/1 -> 2*g/1
  2*g/1 -> Math Function/1
  az_1*Sn/1 -> Product/1
  Math Function/1 -> Product/2
  h_1/1 -> Sum1/1
  Product/1 -> Q_13/1  "Q_13"
  h_3/1 -> Sum1/2

== system Example_Faulty_DataGen/3-Tank-System/Tank 1/Leck in Tank 1 ==
  h_1 : Inport
  2*g1 : Gain  Gain=2*g  SaturateOnIntegerOverflow=on  OutDataTypeStr=Inherit: Same as input  ParamDataTypeStr=Inherit: Same as input
  Math Function1 : Math  Operator=sqrt  SignedPower=on
  az_1*Sl : Gain  Gain=az1*Sl  SaturateOnIntegerOverflow=on  OutDataTypeStr=Inherit: Same as input  ParamDataTypeStr=Inherit: Same as input
  Q_1L : Outport  VectorParamsAs1DForOutWhenUnconnected=off
  wires:
  Math Function1/1 -> az_1*Sl/1
  2*g1/1 -> Math Function1/1
  h_1/1 -> 2*g1/1
  az_1*Sl/1 -> Q_1L/1  "Q_1L"

== system Example_Faulty_DataGen/3-Tank-System/Tank 2/Leck in Tank 2 ==
  h_2 : Inport
  2*g1 : Gain  Gain=2*g  SaturateOnIntegerOverflow=on  OutDataTypeStr=Inherit: Same as input  ParamDataTypeStr=Inherit: Same as input
  Math Function1 : Math  Operator=sqrt  SignedPower=on
  az_2*Sn : Gain  Gain=az2*Sl  SaturateOnIntegerOverflow=on  OutDataTypeStr=Inherit: Same as input  ParamDataTypeStr=Inherit: Same as input
  Q_2L : Outport  VectorParamsAs1DForOutWhenUnconnected=off
  wires:
  Math Function1/1 -> az_2*Sn/1
  2*g1/1 -> Math Function1/1
  h_2/1 -> 2*g1/1
  az_2*Sn/1 -> Q_2L/1  "Q_2L"

== system Example_Faulty_DataGen/3-Tank-System/Tank 2/Zufluss von Tank 3 ==
  h_1 : Inport
  h_3 : Inport  Port=2
  2*g : Gain  Gain=2*g  SaturateOnIntegerOverflow=on  OutDataTypeStr=Inherit: Same as input  ParamDataTypeStr=Inherit: Same as input
  Abs : Abs
  Math Function : Math  Operator=sqrt  SignedPower=on
  Product : Product  SaturateOnIntegerOverflow=on  OutDataTypeStr=Inherit: Same as first input
  Sign : Signum
  Sum1 : Sum  Inputs=-+  SaturateOnIntegerOverflow=on
  az_3*Sn : Gain  Gain=az3*Sn  SaturateOnIntegerOverflow=on  OutDataTypeStr=Inherit: Same as input  ParamDataTypeStr=Inherit: Same as input
  Q_32 : Outport  VectorParamsAs1DForOutWhenUnconnected=off
  wires:
  Sum1/1 -> Sign/1, Abs/1  "h_3-h_2"
  Sign/1 -> az_3*Sn/1
  Abs/1 -> 2*g/1
  2*g/1 -> Math Function/1
  az_3*Sn/1 -> Product/1
  Math Function/1 -> Product/2
  h_1/1 -> Sum1/1
  h_3/1 -> Sum1/2
  Product/1 -> Q_32/1  "Q_32"

== system Example_Faulty_DataGen/3-Tank-System/Tank 2/nom. Ausfluss ==
  h_2 : Inport
  2*g1 : Gain  Gain=2*g  SaturateOnIntegerOverflow=on  OutDataTypeStr=Inherit: Same as input  ParamDataTypeStr=Inherit: Same as input
  Math Function1 : Math  Operator=sqrt  SignedPower=on
  az_2*Sn : Gain  Gain=az2*Sn  SaturateOnIntegerOverflow=on  OutDataTypeStr=Inherit: Same as input  ParamDataTypeStr=Inherit: Same as input
  Q_20 : Outport  VectorParamsAs1DForOutWhenUnconnected=off
  wires:
  Math Function1/1 -> az_2*Sn/1
  2*g1/1 -> Math Function1/1
  h_2/1 -> 2*g1/1
  az_2*Sn/1 -> Q_20/1  "Q_20"

== system Example_Faulty_DataGen/3-Tank-System/Tank 3/Abfluss in Tank 2 ==
  h_2 : Inport
  h_3 : Inport  Port=2
  2*g1 : Gain  Gain=2*g  SaturateOnIntegerOverflow=on  OutDataTypeStr=Inherit: Same as input  ParamDataTypeStr=Inherit: Same as input
  Abs1 : Abs
  Math Function1 : Math  Operator=sqrt  SignedPower=on
  Product1 : Product  SaturateOnIntegerOverflow=on  OutDataTypeStr=Inherit: Same as first input
  Sign1 : Signum
  Sum2 : Sum  Inputs=-+  SaturateOnIntegerOverflow=on
  az_3*Sn1 : Gain  Gain=az3*Sn  SaturateOnIntegerOverflow=on  OutDataTypeStr=Inherit: Same as input  ParamDataTypeStr=Inherit: Same as input
  Q_32 : Outport  VectorParamsAs1DForOutWhenUnconnected=off
  wires:
  Sum2/1 -> Sign1/1, Abs1/1  "h_3-h_2"
  Sign1/1 -> az_3*Sn1/1
  Abs1/1 -> 2*g1/1
  2*g1/1 -> Math Function1/1
  az_3*Sn1/1 -> Product1/1
  Math Function1/1 -> Product1/2
  h_3/1 -> Sum2/2
  h_2/1 -> Sum2/1
  Product1/1 -> Q_32/1  "Q_32"

== system Example_Faulty_DataGen/3-Tank-System/Tank 3/Leck in Tank 3 ==
  h_3 : Inport
  2*g1 : Gain  Gain=2*g  SaturateOnIntegerOverflow=on  OutDataTypeStr=Inherit: Same as input  ParamDataTypeStr=Inherit: Same as input
  Math Function1 : Math  Operator=sqrt  SignedPower=on
  az_3*Sl : Gain  Gain=az3*Sl  SaturateOnIntegerOverflow=on  OutDataTypeStr=Inherit: Same as input  ParamDataTypeStr=Inherit: Same as input
  Q_3L : Outport  VectorParamsAs1DForOutWhenUnconnected=off
  wires:
  Math Function1/1 -> az_3*Sl/1
  2*g1/1 -> Math Function1/1
  h_3/1 -> 2*g1/1
  az_3*Sl/1 -> Q_3L/1  "Q_3L"

== system Example_Faulty_DataGen/3-Tank-System/Tank 3/Zufluss von Tank 1 ==
  h_3 : Inport
  h_1 : Inport  Port=2
  2*g : Gain  Gain=2*g  SaturateOnIntegerOverflow=on  OutDataTypeStr=Inherit: Same as input  ParamDataTypeStr=Inherit: Same as input
  Abs : Abs
  Math Function : Math  Operator=sqrt  SignedPower=on
  Product : Product  SaturateOnIntegerOverflow=on  OutDataTypeStr=Inherit: Same as first input
  Sign : Signum
  Sum1 : Sum  Inputs=-+  SaturateOnIntegerOverflow=on
  az_1*Sn : Gain  Gain=az1*Sn  SaturateOnIntegerOverflow=on  OutDataTypeStr=Inherit: Same as input  ParamDataTypeStr=Inherit: Same as input
  Q_13 : Outport  VectorParamsAs1DForOutWhenUnconnected=off
  wires:
  Sum1/1 -> Sign/1, Abs/1  "h_1-h_3"
  Sign/1 -> az_1*Sn/1
  Abs/1 -> 2*g/1
  2*g/1 -> Math Function/1
  az_1*Sn/1 -> Product/1
  Math Function/1 -> Product/2
  h_3/1 -> Sum1/1
  h_1/1 -> Sum1/2
  Product/1 -> Q_13/1  "Q_13"

== system Example_Faulty_DataGen/Controller/Matrix F/Abfluss in Tank 2 ==
  h_3 : Inport
  h_2 : Inport  Port=2
  2*g1 : Gain  Gain=2*g  SaturateOnIntegerOverflow=on  OutDataTypeStr=Inherit: Same as input  ParamDataTypeStr=Inherit: Same as input
  Abs1 : Abs
  Math Function1 : Math  Operator=sqrt  SignedPower=on
  Product1 : Product  SaturateOnIntegerOverflow=on  OutDataTypeStr=Inherit: Same as first input
  Sign1 : Signum
  Sum2 : Sum  Inputs=-+  SaturateOnIntegerOverflow=on
  az_3*Sn1 : Gain  Gain=az3*Sn  SaturateOnIntegerOverflow=on  OutDataTypeStr=Inherit: Same as input  ParamDataTypeStr=Inherit: Same as input
  Q_32 : Outport  VectorParamsAs1DForOutWhenUnconnected=off
  wires:
  Sum2/1 -> Sign1/1, Abs1/1  "h_3-h_2"
  Sign1/1 -> az_3*Sn1/1
  Abs1/1 -> 2*g1/1
  2*g1/1 -> Math Function1/1
  az_3*Sn1/1 -> Product1/1
  Math Function1/1 -> Product1/2
  Product1/1 -> Q_32/1  "Q_32"
  h_2/1 -> Sum2/1
  h_3/1 -> Sum2/2

== system Example_Faulty_DataGen/Controller/Matrix F/Abfluss zu Tank 3 ==
  h_1 : Inport
  h_3 : Inport  Port=2
  2*g : Gain  Gain=2*g  SaturateOnIntegerOverflow=on  OutDataTypeStr=Inherit: Same as input  ParamDataTypeStr=Inherit: Same as input
  Abs : Abs
  Math Function : Math  Operator=sqrt  SignedPower=on
  Product : Product  SaturateOnIntegerOverflow=on  OutDataTypeStr=Inherit: Same as first input
  Sign : Signum
  Sum1 : Sum  Inputs=+-  SaturateOnIntegerOverflow=on
  az_1*Sn : Gain  Gain=az1*Sn  SaturateOnIntegerOverflow=on  OutDataTypeStr=Inherit: Same as input  ParamDataTypeStr=Inherit: Same as input
  Q_13 : Outport  VectorParamsAs1DForOutWhenUnconnected=off
  wires:
  Sum1/1 -> Sign/1, Abs/1  "h_1-h_3"
  Sign/1 -> az_1*Sn/1
  Abs/1 -> 2*g/1
  2*g/1 -> Math Function/1
  az_1*Sn/1 -> Product/1
  Math Function/1 -> Product/2
  h_1/1 -> Sum1/1
  Product/1 -> Q_13/1  "Q_13"
  h_3/1 -> Sum1/2

== system Example_Faulty_DataGen/Controller/Matrix F/nom. Ausfluss ==
  h_2 : Inport
  2*g1 : Gain  Gain=2*g  SaturateOnIntegerOverflow=on  OutDataTypeStr=Inherit: Same as input  ParamDataTypeStr=Inherit: Same as input
  Math Function1 : Math  Operator=sqrt  SignedPower=on
  az_2*Sn : Gain  Gain=az2*Sn  SaturateOnIntegerOverflow=on  OutDataTypeStr=Inherit: Same as input  ParamDataTypeStr=Inherit: Same as input
  Q_20 : Outport  VectorParamsAs1DForOutWhenUnconnected=off
  wires:
  Math Function1/1 -> az_2*Sn/1
  2*g1/1 -> Math Function1/1
  h_2/1 -> 2*g1/1
  az_2*Sn/1 -> Q_20/1  "Q_20"

== matlab function Example_Faulty_DataGen/dynary_Attack ==
  data: y_1 input; y1 output; y_2 input; y_3 input; y2 output; y3 output; attack input
function [y1,y2,y3] = fcn(y_1,y_2,y_3,attack)
Alpha=[
10
15
20];

if attack==1
    y1=y_2+Alpha(1);
    y2=y_2+Alpha(2);
    y3=y_3+Alpha(3);
else
    y1=y_1;
    y2=y_2;
    y3=y_3;
end

== matlab function Example_Faulty_DataGen/fealthy_Attack/MATLAB Function ==
  data: attack_time input; t output; t input
function t = fcn(attack_time,t)
if t<attack_time
    t=0;
else
    t=t-attack_time;
    if t<10
        t=t;
        % y1=0.0016*t^5-0.0328*t^4+0.1937*t^3-0.0587*t^2-2.2821*t+0;
        % y2=0.0029*t^5-0.0676*t^4+0.5425*t^3-1.6727*t^2+1.2291*t+0;
        % y3=-0.0131*t^5+0.3214*t^4-2.7807*t^3+10.0412*t^2-13.2229*t+0;
    else
        t=mod(t-10,8);
        t=t+2;
        % y1=0.0016*t^5-0.0328*t^4+0.1937*t^3-0.0587*t^2-2.2821*t+0;
        % y2=0.0029*t^5-0.0676*t^4+0.5425*t^3-1.6727*t^2+1.2291*t+0;
        % y3=-0.0131*t^5+0.3214*t^4-2.7807*t^3+10.0412*t^2-13.2229*t+0;
    end

end
